simulink model "threeservos"
settings: Solver=ode45  StartTime=0.0  StopTime=1  RelTol=1e-3
InitFcn:
  | clear functions
libraries: truetime x1
settings Model: ExtModeTrigMode=oneshot  ExtModeArmWhenConnect=off  ExtModeAutoUpdateStatusClock=off  Creator=anton  LastModifiedBy=anton
settings DataIOCC: SaveFormat=Array  SignalLoggingSaveFormat=ModelDataLogs  ReturnWorkspaceOutputs=off
settings OptimizationCC: BlockReduction=off  BooleanDataType=off  ExpressionDepthLimit=2147483647  LifeSpan=inf  SimCompilerOptimization=Off
settings DebuggingCC: SaveWithParameterizedLinksMsg=none  UnderspecifiedInitializationDetection=Classic  MergeDetectMultiDrivingBlocksExec=none  SignalResolutionControl=TryResolveAllWithWarning  MultiTaskDSMMsg=warning  MultiTaskCondExecSysMsg=none  FcnCallInpInsideContextMsg=Use local settings  StateNameClashWarn=warning  SFUnexpectedBacktrackingDiag=warning  SFNoUnconditionalDefaultTransitionDiag=warning
settings HardwareCC: ProdBitPerPointer=32  ProdLargestAtomicFloat=None  ProdIntDivRoundTo=Undefined  ProdEndianess=Unspecified  ProdWordSize=32  ProdHWDeviceType=32-bit Generic  TargetUnknown=on
settings ModelReferenceCC: PropagateSignalLabelsOutOfModel=off
settings SFSimCC: SimUseLocalCustomCode=off
settings RTWCC: RTWUseLocalCustomCode=off  RTWCompilerOptimization=Off
settings GRTTargetCC: CodeReplacementLibrary=C89/C90 (ANSI)  GeneratePreprocessorConditionals=Disable all  CombineOutputUpdateFcns=off  CPPClassGenCompliant=off  GRTInterface=on

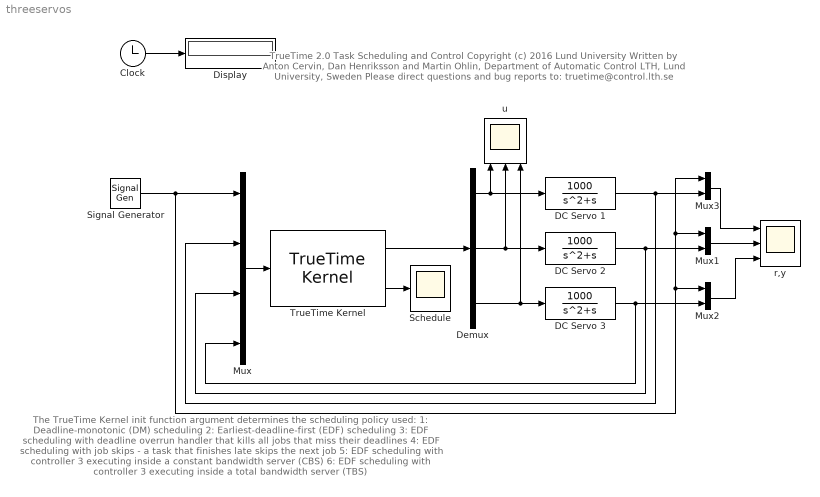
== system threeservos ==
  note: The TrueTime Kernel init function argument determines the scheduling policy used:
      |   1: Deadline-monotonic (DM) scheduling
      |   2: Earliest-deadline-first (EDF) scheduling
      |   3: EDF scheduling with deadline overrun handler that kills all jobs that miss their deadlines
      |   4: EDF scheduling with job skips - a task that finishes late skips the next job
      |   5: EDF scheduling with controller 3 executing inside a constant bandwidth server (CBS)
      |   6: EDF scheduling with controller 3 executing inside a total bandwidth server (TBS)
  note: TrueTime 2.0  Task Scheduling and Control
      | Copyright (c) 2016 Lund University
      | Written by Anton Cervin, Dan Henriksson and Martin Ohlin,
      | Department of Automatic Control LTH, Lund University, Sweden
      | Please direct questions and bug reports to:  truetime@control.lth.se
  Clock : Clock
  DC Servo 1 : TransferFcn  Numerator=[1000]  Denominator=[1 1 0]
  DC Servo 2 : TransferFcn  Numerator=[1000]  Denominator=[1 1 0]
  DC Servo 3 : TransferFcn  Numerator=[1000]  Denominator=[1 1 0]
  Demux : Demux  Outputs=3
  Display : Display
  Mux : Mux
  Mux1 : Mux  Inputs=2
  Mux2 : Mux  Inputs=2
  Mux3 : Mux  Inputs=2
  Schedule : Scope
      settings: TimeRange=1  YMin=1  YMax=3.5  SaveName=ry
  Signal Generator : SignalGenerator  WaveForm=square  Frequency=1.5
  TrueTime Kernel : truetime/TrueTime Kernel  sfun=threeservos_init  args=1  ninputsoutputs=[4 3]  ntriggers=0  trigtype=falling  nwnodenbr=[]  clockoffsetdrift=[0 0]  schedoutput=on  battery=off  poweroutput=off
  r,y : Scope  NumInputPorts=3
      settings: TimeRange=1  YMin=-2~-2~-2  YMax=2~2~2  SaveName=ry1
  u : Scope  NumInputPorts=3
      settings: TimeRange=1  YMin=-2~-5~-5  YMax=2~5~5
  wires:
  Clock/1 -> Display/1
  Signal Generator/1 -> Mux3/1, Mux1/1, Mux2/1, Mux/1
  Demux/2 -> DC Servo 2/1, u/2
  Demux/3 -> DC Servo 3/1, u/3
  DC Servo 1/1 -> Mux3/2, Mux/2
  DC Servo 2/1 -> Mux1/2, Mux/3
  DC Servo 3/1 -> Mux2/2, Mux/4
  Mux2/1 -> r,y/3
  Mux/1 -> TrueTime Kernel/1
  TrueTime Kernel/1 -> Demux/1
  Mux1/1 -> r,y/2
  Mux3/1 -> r,y/1
  Demux/1 -> DC Servo 1/1, u/1
  TrueTime Kernel/2 -> Schedule/1
